simulink library "INT_ASDdc_Governor"  (R2016b)
settings: Solver=VariableStepAuto  StartTime=0.0  StopTime=10.0  RelTol=1e-3
settings Model: Creator=lenovo  LastModifiedBy=lenovo

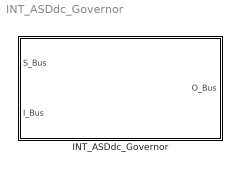
== system INT_ASDdc_Governor ==
  INT_ASDdc_Governor : Subsystem

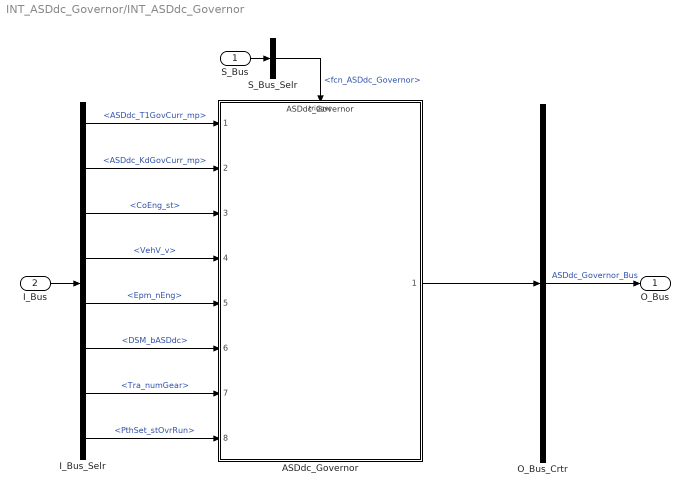
== system INT_ASDdc_Governor/INT_ASDdc_Governor ==
  S_Bus : Inport
  I_Bus : Inport  Port=2
  ASDdc_Governor : ModelReference  ModelNameDialog=ASDdc_Governor  SimulationMode=Normal  ModelReferenceVersion=1.21  TriggerPortName=function  TriggerPortTriggerType=function-call  TriggerPortStatesWhenEnabling=held
  I_Bus_Selr : BusSelector  OutputSignals=ASDdc_T1GovCurr_mp,ASDdc_KdGovCurr_mp,CoEng_st,VehV_v,Epm_nEng,DSM_bASDdc,Tra_numGear,PthSet_stOvrRun
  O_Bus_Crtr : BusCreator  Inputs=1
  S_Bus_Selr : BusSelector  OutputSignals=fcn_ASDdc_Governor
  O_Bus : Outport
  wires:
  S_Bus_Selr/1 -> ASDdc_Governor/Trigger  "<fcn_ASDdc_Governor>"
  S_Bus/1 -> S_Bus_Selr/1
  I_Bus/1 -> I_Bus_Selr/1
  I_Bus_Selr/1 -> ASDdc_Governor/1  "<ASDdc_T1GovCurr_mp>"
  I_Bus_Selr/2 -> ASDdc_Governor/2  "<ASDdc_KdGovCurr_mp>"
  I_Bus_Selr/3 -> ASDdc_Governor/3  "<CoEng_st>"
  I_Bus_Selr/4 -> ASDdc_Governor/4  "<VehV_v>"
  I_Bus_Selr/5 -> ASDdc_Governor/5  "<Epm_nEng>"
  I_Bus_Selr/6 -> ASDdc_Governor/6  "<DSM_bASDdc>"
  I_Bus_Selr/7 -> ASDdc_Governor/7  "<Tra_numGear>"
  I_Bus_Selr/8 -> ASDdc_Governor/8  "<PthSet_stOvrRun>"
  O_Bus_Crtr/1 -> O_Bus/1  "ASDdc_Governor_Bus"
  ASDdc_Governor/1 -> O_Bus_Crtr/1
